simulink model "pfb_fir_generic_async_test_sim4"  (R2012b)
settings: Solver=VariableStepDiscrete  StartTime=0.0  StopTime=10.0  RelTol=1e-3
model workspace (MAT data in the model file):
  synci = [0 1 2 3 4 5 6 7 8 9 10 11 ... (131074 elements, 65537x2)]
  din0 = [0 1 2 3 4 5 6 7 8 9 10 11 ... (16386 elements, 8193x2)]
  din1 = [0 1 2 3 4 5 6 7 8 9 10 11 ... (16386 elements, 8193x2)]
  din2 = [0 1 2 3 4 5 6 7 8 9 10 11 ... (16386 elements, 8193x2)]
  din3 = [0 1 2 3 4 5 6 7 8 9 10 11 ... (16386 elements, 8193x2)]
  din4 = [0 1 2 3 4 5 6 7 8 9 10 11 ... (16386 elements, 8193x2)]
  din5 = [0 1 2 3 4 5 6 7 8 9 10 11 ... (16386 elements, 8193x2)]
  din6 = [0 1 2 3 4 5 6 7 8 9 10 11 ... (16386 elements, 8193x2)]
  din7 = [0 1 2 3 4 5 6 7 8 9 10 11 ... (16386 elements, 8193x2)]
  dvalid = [0 1 2 3 4 5 6 7 8 9 10 11 ... (131072 elements, 65536x2)]
libraries: xbsIndex_r4 x3718, casper_library_delays x1
(part 1 of 18)
settings Model: Creator=andrew  LastModifiedBy=andrew

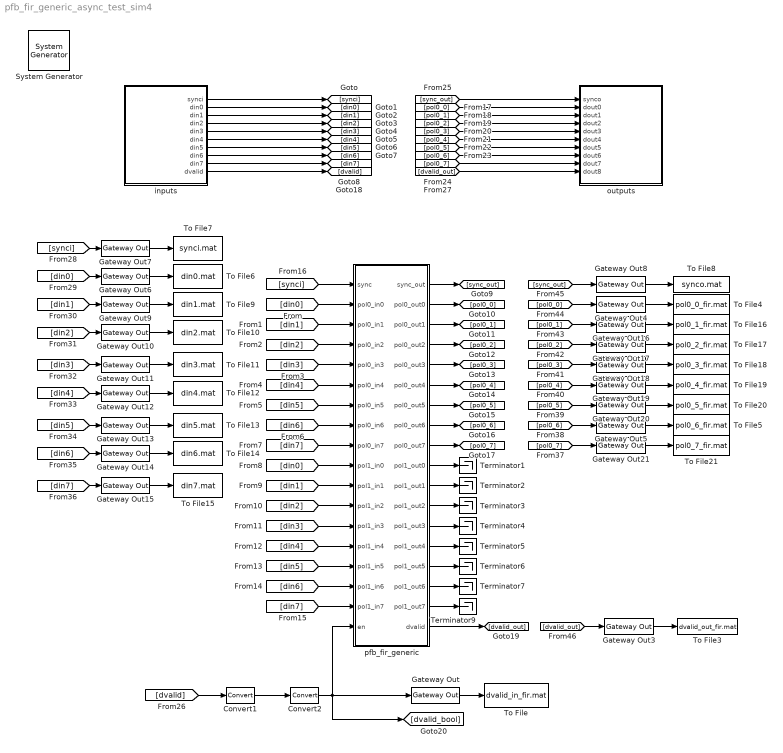
== system pfb_fir_generic_async_test_sim4 ==
  " System Generator" : xbsIndex_r4/ System Generator  Tag=genX  xilinxfamily=Kintex7  part=xc7k325t  speed=-3  package=fbg676  synthesis_tool=XST  clock_wrapper=Clock Enables  directory=./netlist  proj_type=Project Navigator  Synth_file=XST Defaults  Impl_file=ISE Defaults  testbench=off  simulink_period=1  sysclk_period=10  dcm_input_clock_period=10  incr_netlist=off  trim_vbits=Everywhere in SubSystem  dbl_ovrd=According to Block Masks  core_generation=According to Block Masks  run_coregen=off  deprecated_control=off  eval_field=0  block_type=sysgen
  Convert1 : xbsIndex_r4/Convert  gui_display_data_type=Fixed-point  arith_type=Unsigned  n_bits=1  bin_pt=0  float_type=Single  exp_bits=8  fraction_bits=24  quantization="Round  (unbiased: +/- Inf)"  overflow=Saturate  en=off  latency=0  dbl_ovrd=off  pipeline=off  block_type=convert
  Convert2 : xbsIndex_r4/Convert  gui_display_data_type=Boolean  arith_type=Boolean  n_bits=16  bin_pt=14  float_type=Single  exp_bits=8  fraction_bits=24  quantization=Truncate  overflow=Wrap  en=off  latency=0  dbl_ovrd=off  pipeline=off  block_type=convert
  Gateway Out{,3..21} (20 alike) : xbsIndex_r4/Gateway Out  inherit_from_input=off  hdl_port=on  timing_constraint=None  locs_specified=off  LOCs={}  UseAsDAC=off  DACChannel='1'  block_type=gatewayout
  Terminator{1..7,9} (8 alike) : Terminator
  To File : ToFile  Filename=dvalid_in_fir.mat  MatrixName=dvalid_in_fir  SaveFormat=Timeseries
  To File10 : ToFile  Filename=din2.mat  MatrixName=din2_fir  SaveFormat=Timeseries
  To File11 : ToFile  Filename=din3.mat  MatrixName=din3_fir  SaveFormat=Timeseries
  To File12 : ToFile  Filename=din4.mat  MatrixName=din4_fir  SaveFormat=Timeseries
  To File13 : ToFile  Filename=din5.mat  MatrixName=din5_fir  SaveFormat=Timeseries
  To File14 : ToFile  Filename=din6.mat  MatrixName=din6_fir  SaveFormat=Timeseries
  To File15 : ToFile  Filename=din7.mat  MatrixName=din7_fir  SaveFormat=Timeseries
  To File16 : ToFile  Filename=pol0_1_fir.mat  MatrixName=pol0_1_fir  SaveFormat=Timeseries
  To File17 : ToFile  Filename=pol0_2_fir.mat  MatrixName=pol0_2_fir  SaveFormat=Timeseries
  To File18 : ToFile  Filename=pol0_3_fir.mat  MatrixName=pol0_3_fir  SaveFormat=Timeseries
  To File19 : ToFile  Filename=pol0_4_fir.mat  MatrixName=pol0_4_fir  SaveFormat=Timeseries
  To File20 : ToFile  Filename=pol0_5_fir.mat  MatrixName=pol0_5_fir  SaveFormat=Timeseries
  To File21 : ToFile  Filename=pol0_7_fir.mat  MatrixName=pol0_7_fir  SaveFormat=Timeseries
  To File3 : ToFile  Filename=dvalid_out_fir.mat  MatrixName=dvalid_out_fir  SaveFormat=Timeseries
  To File4 : ToFile  Filename=pol0_0_fir.mat  MatrixName=pol0_0_fir  SaveFormat=Timeseries
  To File5 : ToFile  Filename=pol0_6_fir.mat  MatrixName=pol0_6_fir  SaveFormat=Timeseries
  To File6 : ToFile  Filename=din0.mat  MatrixName=din0_fir  SaveFormat=Timeseries
  To File7 : ToFile  Filename=synci.mat  MatrixName=synci_fir  SaveFormat=Timeseries
  To File8 : ToFile  Filename=synco.mat  MatrixName=synco_fir  SaveFormat=Timeseries
  To File9 : ToFile  Filename=din1.mat  MatrixName=din1_fir  SaveFormat=Timeseries
  inputs : Subsystem
  outputs : Subsystem
  pfb_fir_generic : Subsystem  Tag=casper:pfb_fir_generic  AncestorBlock=casper_library_pfbs/pfb_fir_generic  mask(pfb_fir_generic){n_streams=2, PFBSize=13, TotalTaps=8, WindowType=hamming, n_inputs=3, BitWidthIn=10, BitWidthOut=18, CoeffBitWidth=18, complex=off, async=on, add_latency=6, mult_latency=8, bram_latency=8, fan_latency=9, conv_latency=6, quantization=Round  (unbiased: +/- Inf), fwidth=1, coeffs_bram_optimization=Speed, delays_bram_optimization=Speed}
      mask prompts: n_streams "Number input streams?"; PFBSize "Size of PFB: (2^? pnts)"; TotalTaps "Total Number of Taps:"; WindowType "Windowing Function:"; n_inputs "Number of Simultaneous Inputs: (2^?)"; BitWidthIn "Input Bitwidth:"; BitWidthOut "Output Bitwidth:"; CoeffBitWidth "Coefficient Bitwidth:"; complex "Complex data inputs"; async "Asynchronous operation"; add_latency "Add Latency"; mult_latency "Mult Latency"; bram_latency "BRAM Latency"; fan_latency "Fanout Latency"; conv_latency "Convert latency"; quantization "Quantization Behavior"; fwidth "Bin Width Scaling (normal=1)"; coeffs_bram_optimization "Coefficient BRAMs optimization"; delays_bram_optimization "Delay BRAMs optimization"
      mask init:
      | pfb_fir_generic_init(gcb, ...
      |     'n_streams', n_streams, ...
      |     'PFBSize', PFBSize, ...
      |     'TotalTaps', TotalTaps, ...
      |     'WindowType', WindowType, ...
      |     'n_inputs', n_inputs, ...
      |     'complex', complex, ...
      |     'BitWidthIn', BitWidthIn, ...
      |     'BitWidthOut', BitWidthOut, ...
      |     'CoeffBitWidth', CoeffBitWidth, ...
      |     'async', async, ...
      |     'add_latency', add_latency, ...
      |     'mult_latency', mult_latency, ...
      |     'bram_latency', bram_latency, ...
      |     'fan_latency', fan_latency, ...
      |     'conv_latency', conv_latency, ...
      |     'quantization', quantization, ...
      |     'fwidth', fwidth, ...
      |     'coeffs_bram_optimization', coeffs_bram_optimization, ...
      |     'delays_bram_optimization', delays_bram_optimization);
      mask Callback TotalTaps:
      | %num_taps = eval(get_param(gcb, 'TotalTaps'));
      | %old_vec = eval(get_param(gcb, 'mult_spec'));
      | 
      | %vec = 2.*ones(1,num_taps);
      | %old_size = length(old_vec);
      | 
      | %if(old_size <= num_taps),
      | %   new_size = old_size;
      | %else,
      | %    new_size = num_taps;
      | %end
      | 
      | %for n = 1:new_size, vec(n) = old_vec(n); end
      | %set_param(gcb, 'mult_spec', mat2str(vec));
      mask TypeOptions WindowType: bartlett | barthannwin | blackman | blackmanharris | bohamwin | chebwin | flattopwin | gausswin | hamming | hann | kaiser | nuttallwin | parzenwin | rectwin | tukeywin | triang | userwindow
      mask TypeOptions quantization: Truncate | Round  (unbiased: +/- Inf) | Round  (unbiased: Even Values)
      mask Callback fwidth:
      | %num_taps = eval(get_param(gcb, 'TotalTaps'));
      | %old_vec = eval(get_param(gcb, 'mult_spec'));
      | 
      | %vec = 2.*ones(1,num_taps);
      | %old_size = length(old_vec);
      | 
      | %if(old_size <= num_taps),
      | %    new_size = old_size;
      | %else,
      | %    new_size = num_taps;
      | %end
      | 
      | %for n = 1:new_size, vec(n) = old_vec(n); end
      | %set_param(gcb, 'mult_spec', mat2str(vec));
      mask TypeOptions coeffs_bram_optimization: Area | Speed
      mask TypeOptions delays_bram_optimization: Area | Speed
  wires:
  inputs/1(synci) -> [synci]
  inputs/2(din0) -> [din0]
  inputs/3(din1) -> [din1]
  inputs/4(din2) -> [din2]
  inputs/5(din3) -> [din3]
  inputs/6(din4) -> [din4]
  inputs/7(din5) -> [din5]
  inputs/8(din6) -> [din6]
  inputs/9(din7) -> [din7]
  [pol0_7] -> outputs/9(dout7)
  [pol0_6] -> outputs/8(dout6)
  [pol0_5] -> outputs/7(dout5)
  [pol0_4] -> outputs/6(dout4)
  [pol0_3] -> outputs/5(dout3)
  [pol0_2] -> outputs/4(dout2)
  [pol0_1] -> outputs/3(dout1)
  [pol0_0] -> outputs/2(dout0)
  [sync_out] -> outputs/1(synco)
  pfb_fir_generic/10(pol1_out0) -> Terminator1/1
  pfb_fir_generic/11(pol1_out1) -> Terminator2/1
  pfb_fir_generic/12(pol1_out2) -> Terminator3/1
  pfb_fir_generic/13(pol1_out3) -> Terminator4/1
  pfb_fir_generic/14(pol1_out4) -> Terminator5/1
  pfb_fir_generic/15(pol1_out5) -> Terminator6/1
  pfb_fir_generic/16(pol1_out6) -> Terminator7/1
  pfb_fir_generic/18(dvalid) -> [dvalid_out]
  [din0] -> pfb_fir_generic/2(pol0_in0)
  [din1] -> pfb_fir_generic/3(pol0_in1)
  [din2] -> pfb_fir_generic/4(pol0_in2)
  [din3] -> pfb_fir_generic/5(pol0_in3)
  [din4] -> pfb_fir_generic/6(pol0_in4)
  [din5] -> pfb_fir_generic/7(pol0_in5)
  [din6] -> pfb_fir_generic/8(pol0_in6)
  [din7] -> pfb_fir_generic/9(pol0_in7)
  [din0] -> pfb_fir_generic/10(pol1_in0)
  [din1] -> pfb_fir_generic/11(pol1_in1)
  [din2] -> pfb_fir_generic/12(pol1_in2)
  [din3] -> pfb_fir_generic/13(pol1_in3)
  [din4] -> pfb_fir_generic/14(pol1_in4)
  [din5] -> pfb_fir_generic/15(pol1_in5)
  [din6] -> pfb_fir_generic/16(pol1_in6)
  [din7] -> pfb_fir_generic/17(pol1_in7)
  [synci] -> pfb_fir_generic/1(sync)
  pfb_fir_generic/9(pol0_out7) -> [pol0_7]
  pfb_fir_generic/8(pol0_out6) -> [pol0_6]
  pfb_fir_generic/7(pol0_out5) -> [pol0_5]
  pfb_fir_generic/6(pol0_out4) -> [pol0_4]
  pfb_fir_generic/5(pol0_out3) -> [pol0_3]
  pfb_fir_generic/4(pol0_out2) -> [pol0_2]
  pfb_fir_generic/3(pol0_out1) -> [pol0_1]
  pfb_fir_generic/2(pol0_out0) -> [pol0_0]
  pfb_fir_generic/1(sync_out) -> [sync_out]
  pfb_fir_generic/17(pol1_out7) -> Terminator9/1
  inputs/10(dvalid) -> [dvalid]
  [dvalid] -> Convert1/1
  Convert1/1 -> Convert2/1
  Convert2/1 -> [dvalid_bool], pfb_fir_generic/18(en), Gateway Out/1
  Gateway Out/1 -> To File/1
  Gateway Out3/1 -> To File3/1
  [dvalid_out] -> outputs/10(dout8)
  Gateway Out4/1 -> To File4/1
  Gateway Out6/1 -> To File6/1
  Gateway Out7/1 -> To File7/1
  Gateway Out8/1 -> To File8/1
  Gateway Out9/1 -> To File9/1
  Gateway Out10/1 -> To File10/1
  Gateway Out11/1 -> To File11/1
  Gateway Out12/1 -> To File12/1
  Gateway Out13/1 -> To File13/1
  Gateway Out14/1 -> To File14/1
  Gateway Out15/1 -> To File15/1
  [synci] -> Gateway Out7/1
  [din0] -> Gateway Out6/1
  [din1] -> Gateway Out9/1
  [din2] -> Gateway Out10/1
  [din3] -> Gateway Out11/1
  [din4] -> Gateway Out12/1
  [din5] -> Gateway Out13/1
  [din6] -> Gateway Out14/1
  [din7] -> Gateway Out15/1
  Gateway Out16/1 -> To File16/1
  Gateway Out17/1 -> To File17/1
  Gateway Out18/1 -> To File18/1
  Gateway Out19/1 -> To File19/1
  Gateway Out20/1 -> To File20/1
  Gateway Out5/1 -> To File5/1
  Gateway Out21/1 -> To File21/1
  [pol0_7] -> Gateway Out21/1
  [pol0_6] -> Gateway Out5/1
  [pol0_5] -> Gateway Out20/1
  [pol0_4] -> Gateway Out19/1
  [pol0_3] -> Gateway Out18/1
  [pol0_2] -> Gateway Out17/1
  [pol0_1] -> Gateway Out16/1
  [pol0_0] -> Gateway Out4/1
  [sync_out] -> Gateway Out8/1
  [dvalid_out] -> Gateway Out3/1
